simulink model "Predefined_with_GroundTruth"  (R2021b)
settings: Solver=FixedStepAuto  StartTime=0.0  StopTime=stopTime  RelTol=1e-3
model workspace (MAT data in the model file):
  firstWarning = 1
  originalScenarioChecksum = '114339432DE22364D47BB28FC96DC10C'
undefined symbols (not defined in the file): planner_wpts, stopSign_ID, TL_ID, Ts
libraries: drivingscenarioandsensors x2
settings Model: Creator=akshran  LastModifiedBy=moham

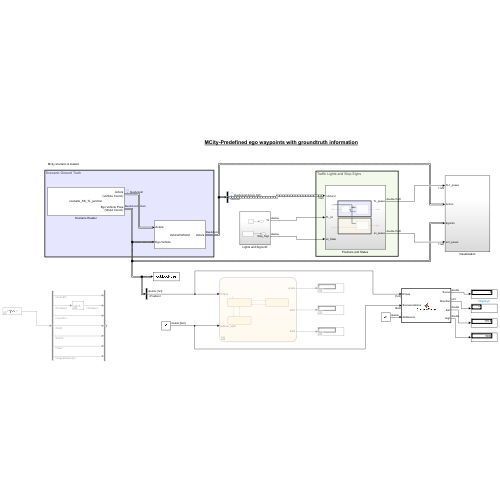
[thumbnail: Simulink's stored preview of the top-level diagram]
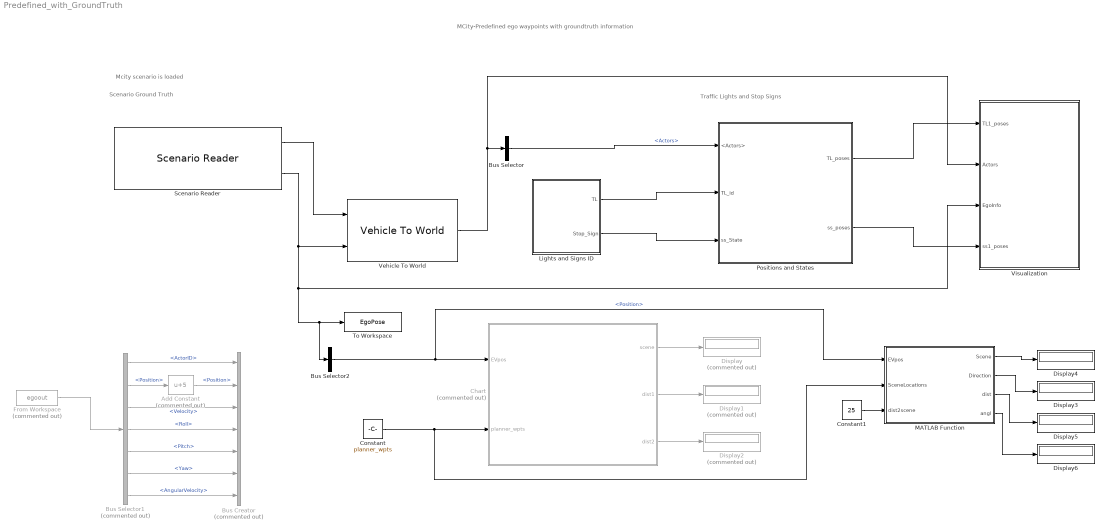
== system Predefined_with_GroundTruth ==
  note: Mcity scenario is loaded
  note: MCity-Predefined ego waypoints with groundtruth information
  note: Traffic Lights and Stop Signs
  note: Scenario Ground Truth
  Add Constant : Bias  Commented=on  Bias=5
  Bus Creator : BusCreator  Commented=on  Inputs=7  OutDataTypeStr=Bus: egoout_bus
  Bus Selector : BusSelector  OutputSignals=Actors
  Bus Selector1 : BusSelector  Commented=on  OutputSignals=ActorID,Position,Velocity,Roll,Pitch,Yaw,AngularVelocity
  Bus Selector2 : BusSelector  OutputSignals=Position
  Chart : Stateflow chart  Commented=on  TreatAsAtomicUnit=on
  Constant : Constant  Value=planner_wpts  VectorParams1D=off
  Constant1 : Constant  Value=25
  Display : Display  Commented=on
  Display1 : Display  Commented=on
  Display2 : Display  Commented=on
  Display{3..6} (4 alike) : Display
  From Workspace : FromWorkspace  Commented=on  VariableName=egoout  OutDataTypeStr=Bus: egoout_bus  SampleTime=Ts
  Lights and Signs ID : Subsystem
  MATLAB Function : MATLAB Function  TreatAsAtomicUnit=on
  "Positions and States " : Subsystem
  Scenario Reader : drivingscenarioandsensors/Scenario Reader  ScenarioSource=From file  ScenarioFileName=C:\Users\moham\MATLAB Drive\AutoDrive Challenge II\ad2_y1_simulationpkg_(2)\ad2_y1_simulationpkg\scenarios\scenario_SS_TL_junction.mat  ScenarioVariableName=scenario  OutputCoordinateSystem=Vehicle coordinates  EgoVehicleSource=Scenario  EgoVehicleActorID=1  OrientVehiclesOnRoad=on  OutputEgoVehiclePose=on  OutputEgoVehicleState=off  SampleTime=Ts  LaneBoundaryOutput=None  LaneBoundaryDistance=0:0.5:9.5  LaneBoundaryLocation=Center of lane markings  BusNameSource=Auto  BusName=BusActors  BusNumActorsSource=Scenario  BusNumActors=100  BusName2Source=Auto  BusName2=BusLaneBoundaries  BusNumLaneBoundariesSource=Scenario  BusNumLaneBoundaries=10  BusName3Source=Auto  BusName3=BusEgoActor  BusName4Source=Auto  BusName4=BusEgoState  ShowCoordinateLabels=on  SimulateUsing=Interpreted execution
  To Workspace : ToWorkspace  VariableName=EgoPose  SaveFormat=Timeseries  SampleTime=-1
  Vehicle To World : drivingscenarioandsensors/Vehicle To World  BusNameSource=Auto  BusName=BusVehicleToWorldActors  SimulateUsing=Interpreted execution
      settings: SourceProductBaseCode=DR
  Visualization : Subsystem
  wires:
  "Positions and States "/1(TL_poses) -> Visualization/1(TL1_poses)
  "Positions and States "/2(ss_poses) -> Visualization/4(ss1_poses)
  Lights and Signs ID/2(Stop_Sign) -> "Positions and States "/3(ss_State)
  Vehicle To World/1 -> Visualization/2(Actors), Bus Selector/1
  Scenario Reader/2 -> Vehicle To World/2, Bus Selector2/1, To Workspace/1, Visualization/3(EgoInfo)
  Bus Selector/1 -> "Positions and States "/1(<Actors>)  "<Actors>"
  Lights and Signs ID/1(TL) -> "Positions and States "/2(TL_id)
  Scenario Reader/1 -> Vehicle To World/1
  From Workspace/1 -> Bus Selector1/1
  Bus Selector1/2 -> Add Constant/1  "<Position>"
  Bus Selector1/1 -> Bus Creator/1  "<ActorID>"
  Bus Selector1/3 -> Bus Creator/3  "<Velocity>"
  Bus Selector1/4 -> Bus Creator/4  "<Roll>"
  Bus Selector1/5 -> Bus Creator/5  "<Pitch>"
  Bus Selector1/6 -> Bus Creator/6  "<Yaw>"
  Bus Selector1/7 -> Bus Creator/7  "<AngularVelocity>"
  Add Constant/1 -> Bus Creator/2  "<Position>"
  Chart/1(scene) -> Display/1
  Bus Selector2/1 -> Chart/1(EVpos), MATLAB Function/1(EVpos)  "<Position>"
  Constant/1 -> Chart/2(planner_wpts), MATLAB Function/2(SceneLocations)
  Chart/2(dist1) -> Display1/1
  Chart/3(dist2) -> Display2/1
  MATLAB Function/2(Direction) -> Display3/1
  MATLAB Function/1(Scene) -> Display4/1
  Constant1/1 -> MATLAB Function/3(dist2scene)
  MATLAB Function/3(dist) -> Display5/1
  MATLAB Function/4(angl) -> Display6/1

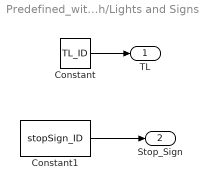
== system Predefined_with_GroundTruth/Lights and Signs ID ==
  Constant : Constant  Value=TL_ID
  Constant1 : Constant  Value=stopSign_ID
  TL : Outport
  Stop_Sign : Outport  Port=2
  wires:
  Constant/1 -> TL/1
  Constant1/1 -> Stop_Sign/1

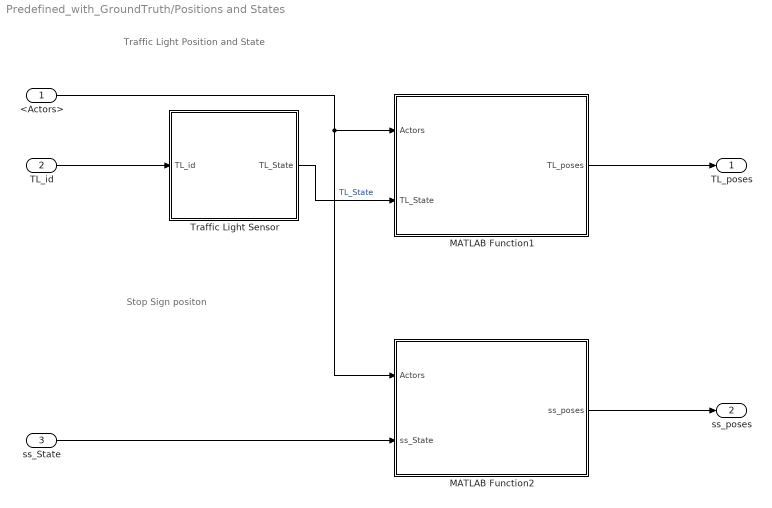
== system Predefined_with_GroundTruth/Positions and States  ==
  note: Stop Sign positon
  note: Traffic Light Position and State
  <Actors> : Inport
  TL_id : Inport  Port=2
  ss_State : Inport  Port=3
  MATLAB Function1 : MATLAB Function  TreatAsAtomicUnit=on
  MATLAB Function2 : MATLAB Function  TreatAsAtomicUnit=on
  Traffic Light Sensor : Subsystem  mask{TrafficLightSensorModeSelection=Cycle}
      mask prompts: TrafficLightSensorModeSelection "Traffic Light Sensor Mode:"
      mask TypeOptions TrafficLightSensorModeSelection: Steady Green | Steady Red | Cycle
      mask DialogControl DescTextVar Prompt: Simulate a traffic light sensor.
  TL_poses : Outport
  ss_poses : Outport  Port=2
  wires:
  <Actors>/1 -> MATLAB Function2/1(Actors), MATLAB Function1/1(Actors)
  ss_State/1 -> MATLAB Function2/2(ss_State)
  TL_id/1 -> Traffic Light Sensor/1(TL_id)
  Traffic Light Sensor/1(TL_State) -> MATLAB Function1/2(TL_State)  "TL_State"
  MATLAB Function2/1(ss_poses) -> ss_poses/1
  MATLAB Function1/1(TL_poses) -> TL_poses/1

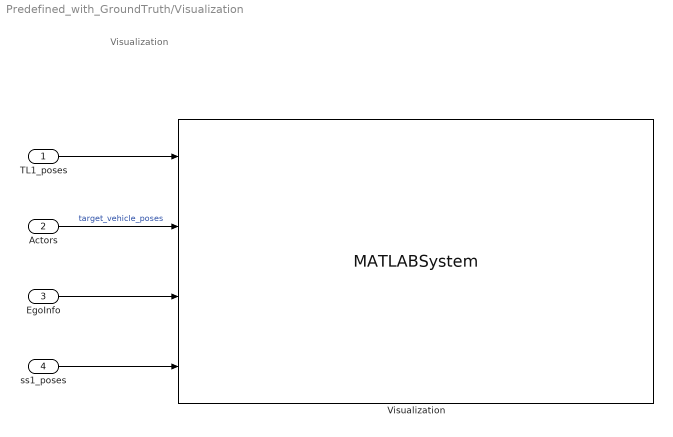
== system Predefined_with_GroundTruth/Visualization ==
  note: Visualization
  TL1_poses : Inport
  Actors : Inport  Port=2
  EgoInfo : Inport  Port=3
  ss1_poses : Inport  Port=4
  Visualization : MATLABSystem  System=TL_vis
      mask Type: TL_vis
      mask Display:
      | disp('TL_vis');
      | port_label('input',1,'TL');
      | port_label('input',2,'TargetPoses');
      | port_label('input',3,'EgoInfo');
      | port_label('input',4,'SS');
  wires:
  EgoInfo/1 -> Visualization/3
  Actors/1 -> Visualization/2  "target_vehicle_poses"
  TL1_poses/1 -> Visualization/1
  ss1_poses/1 -> Visualization/4

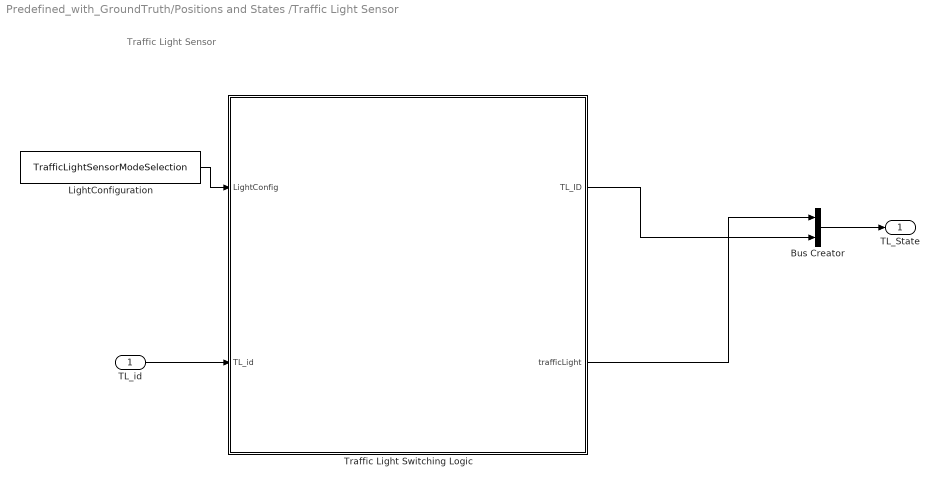
== system Predefined_with_GroundTruth/Positions and States /Traffic Light Sensor ==
  note: Traffic Light Sensor
  TL_id : Inport
  Bus Creator : BusCreator  Inputs=2
  LightConfiguration : Constant  Value=TrafficLightSensorModeSelection
  Traffic Light Switching Logic : Stateflow chart  TreatAsAtomicUnit=on
  TL_State : Outport
  wires:
  LightConfiguration/1 -> Traffic Light Switching Logic/1(LightConfig)
  TL_id/1 -> Traffic Light Switching Logic/2(TL_id)
  Bus Creator/1 -> TL_State/1
  Traffic Light Switching Logic/2(trafficLight) -> Bus Creator/1
  Traffic Light Switching Logic/1(TL_ID) -> Bus Creator/2

== stateflow chart Predefined_with_GroundTruth/Chart ==
  state Check_Scenario
    en,du:
    dist1 = norm(planner_wpts(1,:) - EVpos(1:2));
    dist2 = norm(planner_wpts(2,:) - EVpos(1:2));
    scene = 0;
  state Intersection_4W
    en,du:
    scene = 1;
    dist1 = norm(planner_wpts(1,:) - EVpos(1:2));
    dist2 = norm(planner_wpts(2,:) - EVpos(1:2));
  state Intersection_TL
    en,du:
    scene = 2;
    dist1 = norm(planner_wpts(1,:) - EVpos(1:2));
    dist2 = norm(planner_wpts(2,:) - EVpos(1:2));
  (default) -> Check_Scenario
  Check_Scenario -> Intersection_4W [order 2] : [dist1 < 15]
  Intersection_4W -> Check_Scenario : [dist1 >= 15]
  Check_Scenario -> Intersection_TL [order 1] : [dist2 < 15]
  Intersection_TL -> Check_Scenario : [dist2 >= 15]
  data: EVpos input; scene output; dist1 output; dist2 output; planner_wpts input

== matlab function Predefined_with_GroundTruth/MATLAB Function ==
  data: EVpos input; Scene output; SceneLocations input; Direction output; dist2scene input; dist output; angl output
function [Scene,Direction,dist,angl] = ScenarioFinder(EVpos,SceneLocations,dist2scene)

    % dist = zeros(1,length(SceneLocations));
    for j = 1:length(SceneLocations)
        distXY = SceneLocations(j,:) - EVpos(1:2);
        dist = norm(distXY);

        if (dist <= dist2scene)
            Scene = j;
            angl = atan2d(distXY(2),distXY(1));

            if angl < 0
                angl = angl + 360;
            end

            if (angl > 315) || (angl <= 45) 
                Direction = "N";
            elseif (angl > 225) && (angl <= 315)
                Direction = "E";
            elseif (angl > 135) && (angl <= 225)
                Direction = "S";
            elseif (angl > 45) && (angl <= 135)
                Direction = "W";
            else
                Direction = "Error";
            end
            break
        else
            Scene = 0;
            Direction = " ";
            angl = 1000;
        end

    end

== matlab function Predefined_with_GroundTruth/Positions and States /MATLAB Function2 ==
  data: Actors input; ss_poses output; ss_State input

function ss_poses = findssposes(Actors, ss_State)

n=length(ss_State);
ss_poses=zeros(n,4);
indices=zeros(n,1);
ID=zeros(length(Actors),1);

for i=1:length(Actors)
 ID(i)=Actors(i).ActorID;
end

indices=find(ismember(ID,ss_State));
if(~isempty(indices))
    
    for i=1:n
        ss_poses(i,:)=([Actors(indices(i)).Position(:)',ss_State(i)]);
    end
end

ss_poses(ss_poses==0)=NaN;






% ss1_poses=zeros(1,4);
% ss2_poses=zeros(1,4);
% for i=1:length(Actors)
%     ID=Actors(i).ActorID;
%     
%     if(ID==ss1_State(1))
%         ss1_poses=[Actors(i).Position(:)',ss1_State(1)];
%     elseif ID== (ss1_State(2))
%         ss2_poses=[Actors(i).Position(:)',ss1_State(2)];
%     
%     end
%   
% end
% ss1_poses(ss1_poses==0)=NaN;   
% ss2_poses(ss2_poses==0)=NaN;

== matlab function Predefined_with_GroundTruth/Positions and States /MATLAB Function1 ==
  data: Actors input; TL_poses output; TL_State input

function TL_poses = findTLposes(Actors, TL_State)
n=length(TL_State);
TL_poses=zeros(n/2,5);
indices=zeros(n/2,1);
ID=zeros(length(Actors),1);

for i=1:length(Actors)
 ID(i)=Actors(i).ActorID;
end

indices=find(ismember(ID,TL_State(n/2+1:end)));
if (~isempty(indices))

    for i=1:n/2
        TL_poses(i,:)=([Actors(indices(i)).Position(:)',TL_State(i),ID(indices(i))]);

    end
end
TL_poses(TL_poses==0)=NaN;

== stateflow chart Predefined_with_GroundTruth/Positions and States /Traffic Light Sensor/Traffic Light Switching Logic ==
  state STEADYRED
    entry:
    trafficLight(:)= Red; TL_ID=TL_id;
  state STEADYGREEN
    entry:
    trafficLight(:)= Green; TL_ID=TL_id;
  state START
    entry:
    trafficLight=TL_id;
    trafficLight(:)= Black;TL_ID=TL_id;
  state TRAFFICLIGHT_ODDYELLOW_EVENRED
    entry:
    trafficLight(1:2:end)=Yellow;TL_ID(1:2:end)=TL_id(1:2:end);
    trafficLight(2:2:end) = Red;TL_ID(2:2:end)=TL_id(2:2:end);
  state TRAFFICLIGHT_ODDGREEN_EVENRED
    entry:
    trafficLight(1:2:end)=Green;TL_ID(1:2:end)=TL_id(1:2:end);
    trafficLight(2:2:end) = Red;TL_ID(2:2:end)=TL_id(2:2:end);
  state TRAFFICLIGHT_ODDRED_EVENYELLOW
    entry:
    trafficLight(1:2:end)=Red;TL_ID(1:2:end)=TL_id(1:2:end);
    trafficLight(2:2:end) = Yellow;TL_ID(2:2:end)=TL_id(2:2:end);
  state TRAFFICLIGHT_ODDRED_EVENGREEN
    entry:
    trafficLight(1:2:end)=Red;TL_ID(1:2:end)=TL_id(1:2:end);
    trafficLight(2:2:end) = Green;TL_ID(2:2:end)=TL_id(2:2:end);
  (default) -> START
  START -> STEADYGREEN [order 3] : [LightConfig==1]
  START -> STEADYRED [order 1] : [LightConfig==2]
  START -> TRAFFICLIGHT_ODDGREEN_EVENRED [order 2] : [LightConfig ==3]
  TRAFFICLIGHT_ODDGREEN_EVENRED -> TRAFFICLIGHT_ODDYELLOW_EVENRED : after(0.5,sec)
  TRAFFICLIGHT_ODDYELLOW_EVENRED -> TRAFFICLIGHT_ODDRED_EVENGREEN : after(0.5,sec)
  TRAFFICLIGHT_ODDRED_EVENYELLOW -> TRAFFICLIGHT_ODDGREEN_EVENRED : after(0.5,sec)
  TRAFFICLIGHT_ODDRED_EVENGREEN -> TRAFFICLIGHT_ODDRED_EVENYELLOW : after(0.5,sec)
  data: Green constant double =3; Red constant double =1; Yellow constant double =2; LightConfig input; TL_id input; Black constant double =0; TL_ID output; trafficLight output
